simulink model "zad1"  (R2020b)
settings: Solver=VariableStepAuto  StartTime=0.0  StopTime=10.0  RelTol=1e-3
values from neighbouring files (symbols this model uses):
  Cvg =     [kwpss zad1.m]    (also in kwpss_zad1.m = 400800)
  Cvw = Cpp * dp * Vp    [kwpss zad1.m]    (also in kwpss_zad1.m = 36000)
  dT = 0    [kwpss_zad1.m]
  fmg = pw * fg    [kwpss zad1.m]    (also in kwpss_zad1.m = 0)
  Kcg = qgN/(TgpN - TwewN)    (= 0.1)    [kwpss_zad1.m]
  Kcw = qgN/(TwewN - TzewN)    (= 0.125)    [kwpss_zad1.m]
  Tzew0 = 10    [kwpss_zad1.m]
undefined symbols (not defined in the file or in its folder): cpw, qt
settings Model: Creator=Lab320  LastModifiedBy=Lab320

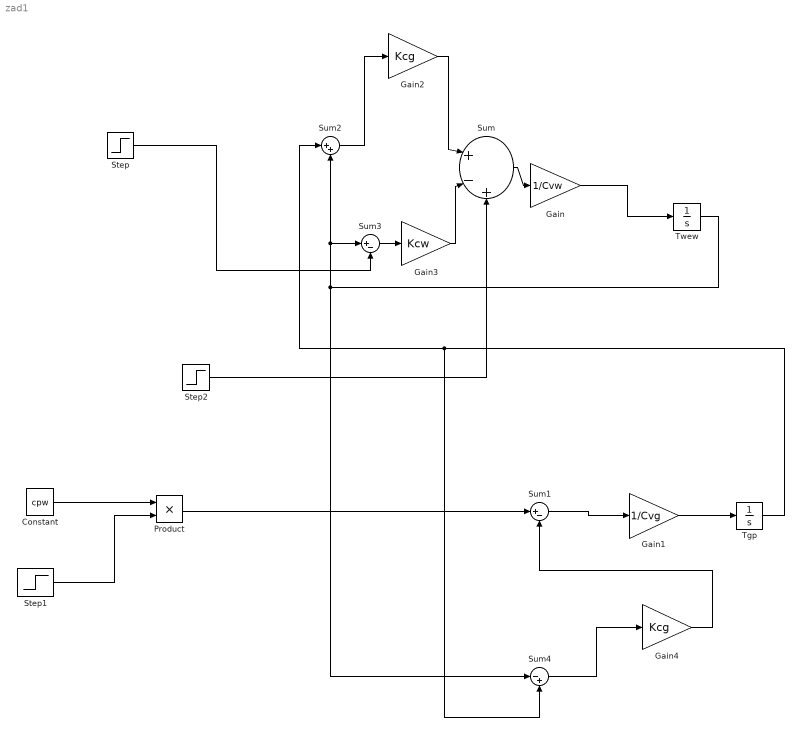
== system zad1 ==
  Constant : Constant  Value=cpw
  Gain : Gain  Gain=1/Cvw
  Gain1 : Gain  Gain=1/Cvg
  Gain2 : Gain  Gain=Kcg
  Gain3 : Gain  Gain=Kcw
  Gain4 : Gain  Gain=Kcg
  Product : Product
  Step : Step  Time=dT  Before=Tzew0  After=Tzew0 + dT  SampleTime=0
  Step1 : Step  Time=dT  Before=fmg  After=fmg + dT  SampleTime=0
  Step2 : Step  Time=dT  Before=qt  After=qt + dT  SampleTime=0
  Sum : Sum  Inputs=|+-+
  Sum1 : Sum  Inputs=|+-
  Sum2 : Sum  Inputs=|++
  Sum3 : Sum  Inputs=|+-
  Sum4 : Sum  Inputs=|-+
  Tgp : Integrator
  Twew : Integrator
  wires:
  Gain/1 -> Twew/1
  Gain1/1 -> Tgp/1
  Sum1/1 -> Gain1/1
  Sum/1 -> Gain/1
  Gain2/1 -> Sum/1
  Gain3/1 -> Sum/2
  Tgp/1 -> Sum2/1, Sum4/2
  Twew/1 -> Sum4/1, Sum3/1, Sum2/2
  Sum2/1 -> Gain2/1
  Sum3/1 -> Gain3/1
  Step/1 -> Sum3/2
  Step2/1 -> Sum/3
  Constant/1 -> Product/1
  Step1/1 -> Product/2
  Product/1 -> Sum1/1
  Gain4/1 -> Sum1/2
  Sum4/1 -> Gain4/1
